simulink model "simulink_filter"  (R2017b)
settings: Solver=FixedStepDiscrete  StartTime=0.0  StopTime=inf  RelTol=1e-3
settings Model: Creator=Heisenberg  LastModifiedBy=Heisenberg
settings SolverCC: AutoInsertRateTranBlk=on
settings DataIOCC: LimitDataPoints=on  SaveOutput=off  SignalLogging=off  DSMLogging=off  SaveTime=off
settings OptimizationCC: LifeSpan=inf
settings DebuggingCC: AlgebraicLoopMsg=error  SingleTaskRateTransMsg=error  AllowSymbolicDim=off  SFUnexpectedBacktrackingDiag=warning  SFNoUnconditionalDefaultTransitionDiag=warning  SFExecutionAtInitializationDiag=none
settings CodeAppCC: StateflowObjectComments=on
settings GRTTargetCC: TargetLangStandard=C89/C90 (ANSI)  GeneratePreprocessorConditionals=Disable all

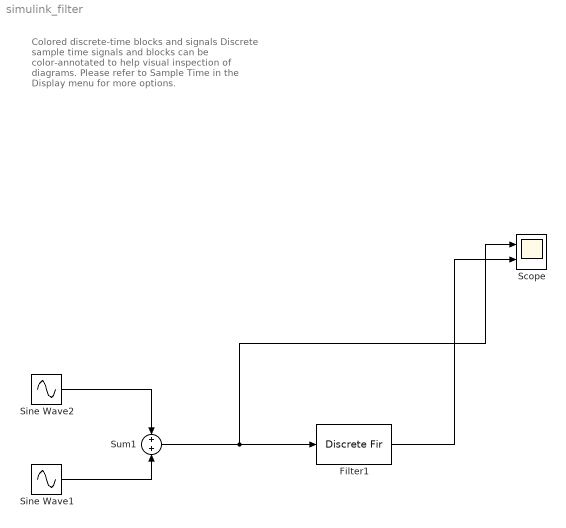
== system simulink_filter ==
  note: Colored discrete-time blocks and signals
      | Discrete sample time signals and blocks can be color-annotated to help visual inspection of diagrams. Please refer to Sample Time in the Display menu for more options.
  Filter1 : DiscreteFir  Tag=BlockMethodSubSystem  Coefficients=[0.00787642536531692888 0.00458035362071161113 -0.0582957276426351381 -0.0844663922503690462 0.1311812688323509 0.451445090848806907 0.451445090848806907 0.1311812688323509 -0.0844663922503690462 -0.0582957276426351381 0.00458035362071161113 0.00787642536531692888]  InputProcessing=Columns as channels (frame based)
  Scope : Scope  NumInputPorts=2
  Sine Wave1 : Sin  Frequency=2*pi*5000  Samples=1  SampleTime=1/8000
  Sine Wave2 : Sin  Frequency=2*pi*50  Samples=1  SampleTime=1/8000
  Sum1 : Sum
  wires:
  Sine Wave1/1 -> Sum1/2
  Sum1/1 -> Scope/1, Filter1/1
  Sine Wave2/1 -> Sum1/1
  Filter1/1 -> Scope/2
